simulink model "inv_pend_damp"  (R2016a)
settings: Solver=VariableStepAuto  StartTime=0.0  StopTime=100  MaxStep=0.01  RelTol=1e-3
InitFcn:
  | init
values from neighbouring files (symbols this model uses):
  b = 1:10    [alg.m]    (also in init.m = 0.1)
  g = 9.8    [init.m]
  J = m*l^2    (= 1)    [init.m]
  l = 1    [init.m]
  m = 1    [init.m]
libraries: simulink_extras x1
settings Model: Creator=roslovetspv  LastModifiedBy=roslovetspv

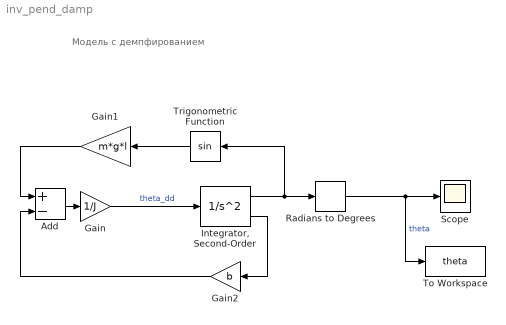
== system inv_pend_damp ==
  note: Модель с демпфированием
  Add : Sum  Inputs=+-
  Gain : Gain  Gain=1/J
  Gain1 : Gain  Gain=m*g*l
  Gain2 : Gain  Gain=b
  "Integrator, Second-Order" : SecondOrderIntegrator  ICX=0.01
  Radians to Degrees : simulink_extras/Transformations/Radians to Degrees
  Scope : Scope
  To Workspace : ToWorkspace  VariableName=theta  SampleTime=-1
  Trigonometric Function : Trigonometry
  wires:
  Radians to Degrees/1 -> To Workspace/1, Scope/1  "theta"
  "Integrator, Second-Order"/1 -> Trigonometric Function/1, Radians to Degrees/1
  Gain/1 -> "Integrator, Second-Order"/1  "theta_dd"
  Trigonometric Function/1 -> Gain1/1
  Gain1/1 -> Add/1
  Add/1 -> Gain/1
  "Integrator, Second-Order"/2 -> Gain2/1
  Gain2/1 -> Add/2
